simulink model "mbd_example_pwm"  (R2022b)
settings: Solver=FixedStepDiscrete  StartTime=0.0  StopTime=10.0  RelTol=1e-3  EnableMultiTasking=on
PostLoadFcn:
  | run([bdroot '_init']);
InitFcn:
  | checkModelFolder; % Optional
  | run([bdroot '_init']);
values from neighbouring files (symbols this model uses):
  T_s_LED1 = 1/LED1_Hz    (= 0.5)    [mbd_example_pwm_init.m]
  T_s_LED2 = 1/LED2_Hz    (= 1)    [mbd_example_pwm_init.m]
libraries: MbdLib_Pwm x14, MbdLib_Digital x11, MbdLib_Timer x5, MbdLib_Sys x4, MbdLib_LpTimer x4, MbdLib_Required x1
settings Model: Creator=KenYoshioka  LastModifiedBy=KenYoshioka
settings SolverCC: AutoInsertRateTranBlk=on
settings OptimizationCC: DefaultParameterBehavior=Inlined  DefaultUnderspecifiedDataType=single  EnhancedBackFolding=on  BooleansAsBitfields=on  PassReuseOutputArgsAs=Individual arguments  ZeroExternalMemoryAtStartup=off  ZeroInternalMemoryAtStartup=off  OptimizeBlockOrder=speed  DifferentSizesBufferReuse=on  EfficientTunableParamExpr=on
settings DebuggingCC: ParameterTunabilityLossMsg=error
settings HardwareCC: ProdBitPerPointer=32  ProdBitPerSizeT=32  ProdBitPerPtrDiffT=32  ProdLargestAtomicInteger=Long  ProdLargestAtomicFloat=Double  ProdWordSize=32  ProdHWDeviceType=ARM Compatible->ARM Cortex-M
settings ModelReferenceCC: EnableRefExpFcnMdlSchedulingChecks=on  ModelReferenceNumInstancesAllowed=Single
settings SFSimCC: MATLABDynamicMemAlloc=off
settings RTWCC: Description=MBD Embedded Target STM32 Cortex M4 (real-time)  SystemTargetFile=MBD_STM32_stf.tlc  TemplateMakefile=MBD_STM32.tmf  Toolchain=arm-none-eabi - v9.3.1
settings CodeAppCC: ForceParamTrailComments=on  IgnoreCustomStorageClasses=off  MaxIdLength=255  OperatorAnnotations=on  SimulinkDataObjDesc=on  SFDataObjDesc=on  InsertBlockDesc=on
settings STFCustomTargetCC: MultiwordLength=256  IncludeMdlTerminateFcn=off  CombineOutputUpdateFcns=on  CombineSignalStateStructs=on  SuppressErrorStatus=on  ERTCustomFileBanners=on  SupportContinuousTime=off  RemoveResetFunc=on  MATLABClassNameForMDSCustomization=Simulink.SoftwareTarget.ERTCustomization  UseToolchainInfoCompliant=on  SystemTargetFile=MBD_STM32_stf.tlc
settings ERTTargetCC: ParMdlRefBuildCompliant=off  CompOptLevelCompliant=off  ConcurrentExecutionCompliant=off  IncludeMdlTerminateFcn=off  CombineSignalStateStructs=on  SuppressErrorStatus=on  SupportNonInlinedSFcns=on  ModelStepFunctionPrototypeControlCompliant=off  CPPClassGenCompliant=off  ExtModeStaticAllocSize=2000  InlinedParameterPlacement=NonHierarchical  ERTCustomFileTemplate=mbd_lib_interface.tlc  MaxLineWidth=110

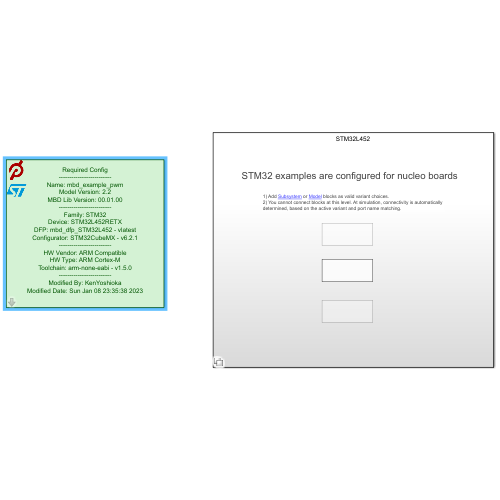
[thumbnail: Simulink's stored preview of the top-level diagram]
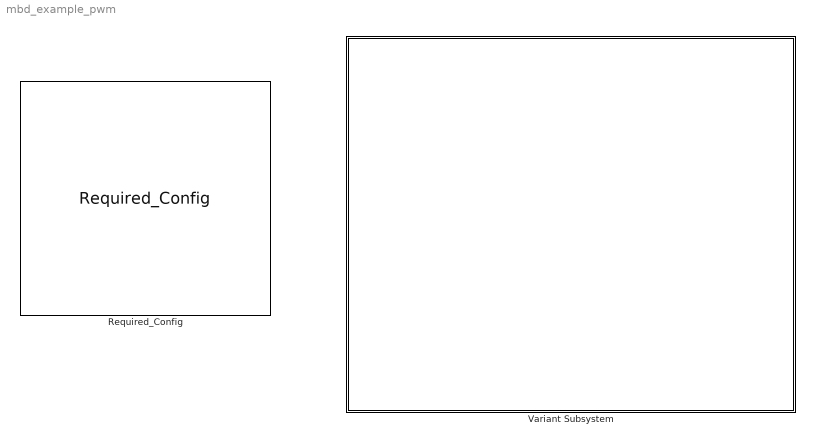
== system mbd_example_pwm ==
  Required_Config : MbdLib_Required/Required_Config  Tag=MBD_Target_Info  Param_update=1
      settings: SourceProductName=Peloton Interface Library
  Variant Subsystem : Subsystem  Variant=on

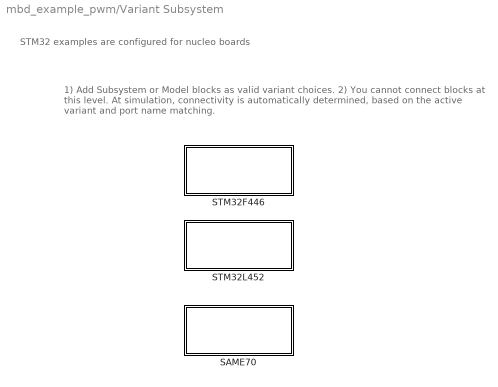
== system mbd_example_pwm/Variant Subsystem ==
  note: 1) Add Subsystem or Model blocks as valid variant choices.
      | 2) You cannot connect blocks at this level. At simulation, connectivity is automatically
      | determined, based on the active variant and port name matching.
  note: STM32 examples are configured for nucleo boards
  SAME70 : Subsystem  VariantControl=VAR_MBD_SAME70
  STM32F446 : Subsystem  VariantControl=VAR_MBD_STM32F446
  STM32L452 : Subsystem  VariantControl=VAR_MBD_STM32L452

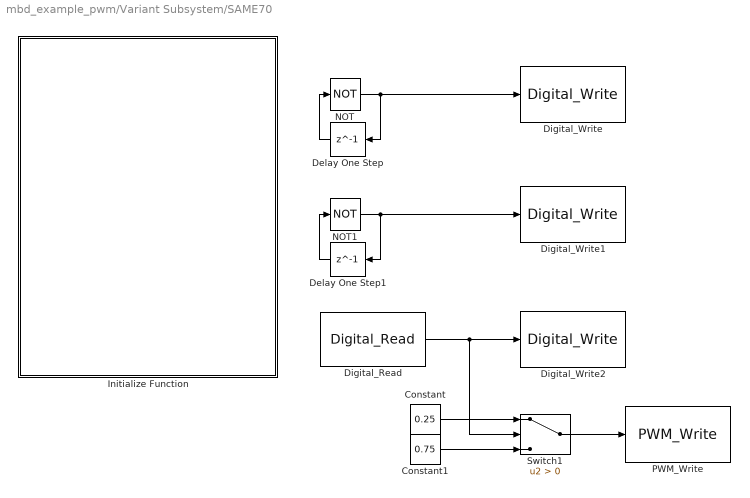
== system mbd_example_pwm/Variant Subsystem/SAME70 ==
  Constant : Constant  Value=0.25
  Constant1 : Constant  Value=0.75
  Delay One Step : Delay  DelayLength=1  SampleTime=T_s_LED1
  Delay One Step1 : Delay  DelayLength=1  SampleTime=T_s_LED2
  Digital_Read : MbdLib_Digital/Digital_Read  Param_module=D  Param_ch=28  Param_sampleTime=-1  Sim_invert=off  Sim_out=0
      settings: SourceProductName=Peloton Interface Library
  Digital_Write : MbdLib_Digital/Digital_Write  Param_module=D  Param_ch=7  Param_sampleTime=-1
      settings: SourceProductName=Peloton Interface Library
  Digital_Write1 : MbdLib_Digital/Digital_Write  Param_module=D  Param_ch=8  Param_sampleTime=-1
      settings: SourceProductName=Peloton Interface Library
  Digital_Write2 : MbdLib_Digital/Digital_Write  Param_module=D  Param_ch=9  Param_sampleTime=-1
      settings: SourceProductName=Peloton Interface Library
  Initialize Function : Subsystem  TreatAsAtomicUnit=on
  NOT : Logic  Operator=NOT  IconShape=distinctive  AllPortsSameDT=off  OutDataTypeStr=boolean
  NOT1 : Logic  Operator=NOT  IconShape=distinctive  AllPortsSameDT=off  OutDataTypeStr=boolean
  PWM_Write : MbdLib_Pwm/PWM_Write  Param_module=0  Param_ch_visible=1  Param_ch=1  Param_sync=off  Param_sampleTime=-1
      settings: SourceProductName=Peloton Interface Library
  Switch1 : Switch  Criteria=u2 > Threshold  SaturateOnIntegerOverflow=off  InputSameDT=off
  wires:
  NOT1/1 -> Digital_Write1/1, Delay One Step1/1
  NOT/1 -> Digital_Write/1, Delay One Step/1
  Delay One Step/1 -> NOT/1
  Delay One Step1/1 -> NOT1/1
  Digital_Read/1 -> Switch1/2, Digital_Write2/1
  Constant/1 -> Switch1/1
  Constant1/1 -> Switch1/3
  Switch1/1 -> PWM_Write/1

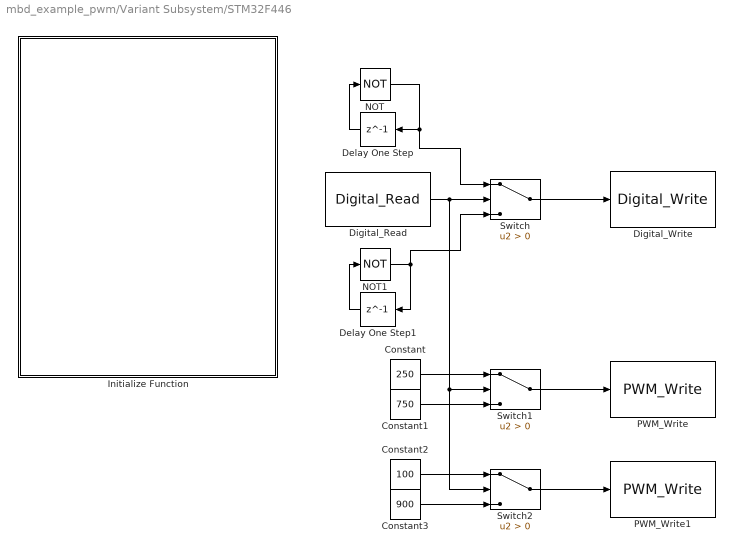
== system mbd_example_pwm/Variant Subsystem/STM32F446 ==
  Constant : Constant  Value=250
  Constant1 : Constant  Value=750
  Constant2 : Constant  Value=100
  Constant3 : Constant  Value=900
  Delay One Step : Delay  DelayLength=1  SampleTime=T_s_LED1
  Delay One Step1 : Delay  DelayLength=1  SampleTime=T_s_LED2
  Digital_Read : MbdLib_Digital/Digital_Read  Param_module=C  Param_ch=13  Param_sampleTime=-1  Sim_invert=off  Sim_out=0
      settings: SourceProductName=Peloton Interface Library
  Digital_Write : MbdLib_Digital/Digital_Write  Param_module=C  Param_ch=10  Param_sampleTime=-1
      settings: SourceProductName=Peloton Interface Library
  Initialize Function : Subsystem  TreatAsAtomicUnit=on
  NOT : Logic  Operator=NOT  IconShape=distinctive  AllPortsSameDT=off  OutDataTypeStr=boolean
  NOT1 : Logic  Operator=NOT  IconShape=distinctive  AllPortsSameDT=off  OutDataTypeStr=boolean
  PWM_Write : MbdLib_Pwm/PWM_Write  Param_module=2  Param_ch_visible=1  Param_ch=1  Param_sync=off  Param_sampleTime=-1
      settings: SourceProductName=Peloton Interface Library
  PWM_Write1 : MbdLib_Pwm/PWM_Write  Param_module=2  Param_ch_visible=2  Param_ch=2  Param_sync=off  Param_sampleTime=-1
      settings: SourceProductName=Peloton Interface Library
  Switch : Switch  Criteria=u2 > Threshold  SaturateOnIntegerOverflow=off  InputSameDT=off
  Switch1 : Switch  Criteria=u2 > Threshold  SaturateOnIntegerOverflow=off  InputSameDT=off
  Switch2 : Switch  Criteria=u2 > Threshold  SaturateOnIntegerOverflow=off  InputSameDT=off
  wires:
  NOT1/1 -> Switch/3, Delay One Step1/1
  NOT/1 -> Switch/1, Delay One Step/1
  Delay One Step/1 -> NOT/1
  Delay One Step1/1 -> NOT1/1
  Switch/1 -> Digital_Write/1
  Switch1/1 -> PWM_Write/1
  Constant/1 -> Switch1/1
  Constant1/1 -> Switch1/3
  Constant2/1 -> Switch2/1
  Constant3/1 -> Switch2/3
  Switch2/1 -> PWM_Write1/1
  Digital_Read/1 -> Switch2/2, Switch1/2, Switch/2

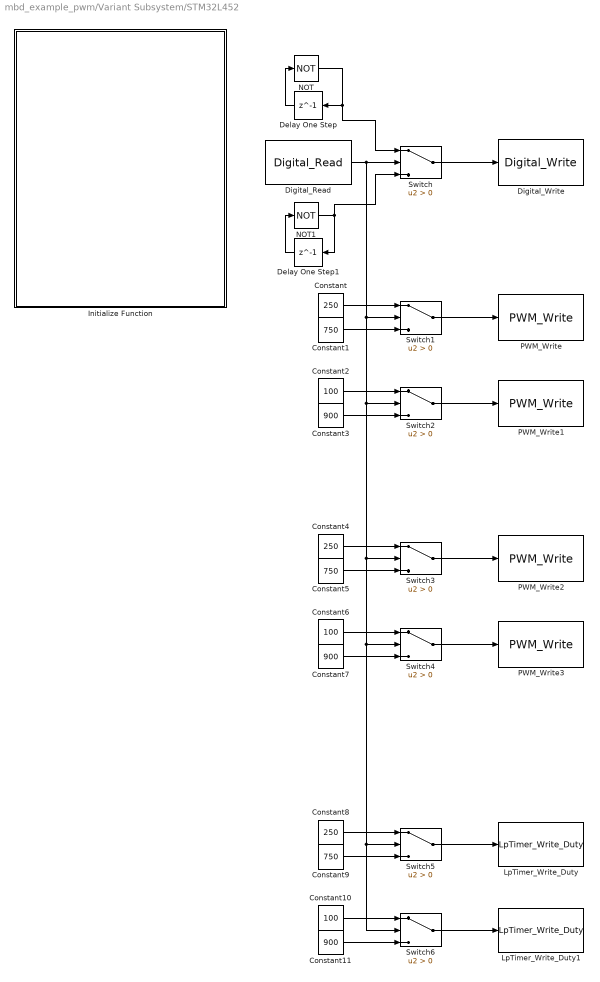
== system mbd_example_pwm/Variant Subsystem/STM32L452 ==
  Constant : Constant  Value=250
  Constant1 : Constant  Value=750
  Constant10 : Constant  Value=100
  Constant11 : Constant  Value=900
  Constant2 : Constant  Value=100
  Constant3 : Constant  Value=900
  Constant4 : Constant  Value=250
  Constant5 : Constant  Value=750
  Constant6 : Constant  Value=100
  Constant7 : Constant  Value=900
  Constant8 : Constant  Value=250
  Constant9 : Constant  Value=750
  Delay One Step : Delay  DelayLength=1  SampleTime=T_s_LED1
  Delay One Step1 : Delay  DelayLength=1  SampleTime=T_s_LED2
  Digital_Read : MbdLib_Digital/Digital_Read  Param_module=C  Param_ch=13  Param_sampleTime=-1  Sim_invert=off  Sim_out=0
      settings: SourceProductName=Peloton Interface Library
  Digital_Write : MbdLib_Digital/Digital_Write  Param_module=C  Param_ch=10  Param_sampleTime=-1
      settings: SourceProductName=Peloton Interface Library
  Initialize Function : Subsystem  TreatAsAtomicUnit=on
  LpTimer_Write_Duty : MbdLib_LpTimer/LpTimer_Write_Duty  Param_module=1  Param_sampleTime=-1
      settings: SourceProductName=Peloton Interface Library
  LpTimer_Write_Duty1 : MbdLib_LpTimer/LpTimer_Write_Duty  Param_module=2  Param_sampleTime=-1
      settings: SourceProductName=Peloton Interface Library
  NOT : Logic  Operator=NOT  IconShape=distinctive  AllPortsSameDT=off  OutDataTypeStr=boolean
  NOT1 : Logic  Operator=NOT  IconShape=distinctive  AllPortsSameDT=off  OutDataTypeStr=boolean
  PWM_Write : MbdLib_Pwm/PWM_Write  Param_module=1  Param_ch_visible=1  Param_ch=1  Param_sync=off  Param_sampleTime=-1
      settings: SourceProductName=Peloton Interface Library
  PWM_Write1 : MbdLib_Pwm/PWM_Write  Param_module=1  Param_ch_visible=2  Param_ch=2  Param_sync=off  Param_sampleTime=-1
      settings: SourceProductName=Peloton Interface Library
  PWM_Write2 : MbdLib_Pwm/PWM_Write  Param_module=2  Param_ch_visible=1  Param_ch=1  Param_sync=off  Param_sampleTime=-1
      settings: SourceProductName=Peloton Interface Library
  PWM_Write3 : MbdLib_Pwm/PWM_Write  Param_module=2  Param_ch_visible=2  Param_ch=2  Param_sync=off  Param_sampleTime=-1
      settings: SourceProductName=Peloton Interface Library
  Switch{,1..6} (7 alike) : Switch  Criteria=u2 > Threshold  SaturateOnIntegerOverflow=off  InputSameDT=off
  wires:
  NOT1/1 -> Switch/3, Delay One Step1/1
  NOT/1 -> Switch/1, Delay One Step/1
  Delay One Step/1 -> NOT/1
  Delay One Step1/1 -> NOT1/1
  Switch/1 -> Digital_Write/1
  Switch1/1 -> PWM_Write/1
  Constant/1 -> Switch1/1
  Constant1/1 -> Switch1/3
  Constant3/1 -> Switch2/3
  Constant2/1 -> Switch2/1
  Switch2/1 -> PWM_Write1/1
  Constant7/1 -> Switch4/3
  Constant6/1 -> Switch4/1
  Constant5/1 -> Switch3/3
  Constant4/1 -> Switch3/1
  Switch3/1 -> PWM_Write2/1
  Switch4/1 -> PWM_Write3/1
  Constant11/1 -> Switch6/3
  Constant8/1 -> Switch5/1
  Constant10/1 -> Switch6/1
  Digital_Read/1 -> Switch6/2, Switch5/2, Switch4/2, Switch3/2, Switch2/2, Switch1/2, Switch/2
  Constant9/1 -> Switch5/3
  Switch5/1 -> LpTimer_Write_Duty/1
  Switch6/1 -> LpTimer_Write_Duty1/1

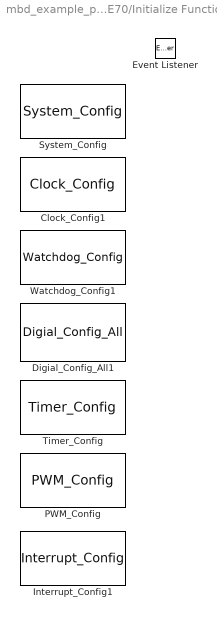
== system mbd_example_pwm/Variant Subsystem/SAME70/Initialize Function ==
  Clock_Config1 : MbdLib_Sys/Clock_Config  Priority=10  Param_frequency=Peripheral_Clock_Hz  Param_priority=10  Param_sampleTime=-1
      settings: AttributesFormatString=priority=%<priority>  SourceProductName=Peloton Interface Library
  Digial_Config_All1 : MbdLib_Digital/Digial_Config_All  Priority=30  Param_channels={ 'A', '0', 'off', '0 : input', '0 : low', '0 : none', '0 : none', '0 : low', '0 : low'; 'A', '1', 'off', '0 : input', '0 : low', '0 : none', '0 : none', '0 : low', '0 : low'; 'A', '2', 'off', '0 : input', '0 : low', '0 : none', '0 : none', '0 : low', '0 : low'; 'A', '3', 'off', '0 : input', '0 : low', '0 : none', '0 : none', '0 : low', '0 : low'; 'A', '4', 'off', '0 : input', '0 : low', '0 : none', '0 : none', '0 : low', '0 : low'; 'A', '5', 'off', '0 : input', '0 : low', '0 : none', '0 : none', '0 : low', '0 : low'; 'A', '6', 'off', '0 : input', '0 : low', '0 : none', '0 : none', '0 : low', '0 : low'; 'A', '7', 'off', '0 : input', '0 : low', '0 : none', '0 : none', '0 : low', '0 : low'; 'A', '8', 'off', '0 : input', '0 : low', '0 : none', '0 : none', '0 : low', '0 : low'; 'A', '9', 'off', '0 : input', '0 : low', '0 : none', '0 : none', '0 : low', '0 : low'; 'A', '10', 'off', '0 : input', '0 : low', '0 : none', '0 : none', '0 : low', '0 : low'; 'A', '11', 'off', '0 : input', '0 : low', '0 : none', '0 : none', '0 : low', '0 : low'; 'A', '12', 'off', '0 : input', '0 : low', '0 : none', '0 : none', '0 : low', '0 : low'; 'A', '13', 'off', '0 : input', '0 : low', '0 : none', '0 : none', '0 : low', '0 : low'; 'A', '14', 'off', '0 : input', '0 : low', '0 : none', '0 : none', '0 : low', '0 : low'; 'A', '15', 'off', '0 : input', '0 : low', '0 : none', '0 : none', '0 : low', '0 : low'; 'A', '16', 'off', '0 : input', '0 : low', '0 : none', '0 : none', '0 : low', '0 : low'; 'A', '17', 'off', '0 : input', '0 : low', '0 : none', '0 : none', '0 : low', '0 : low'; 'A', '18', 'off', '0 : input', '0 : low', '0 : none', '0 : none', '0 : low', '0 : low'; 'A', '19', 'off', '0 : input', '0 : low', '0 : none', '0 : none', '0 : low', '0 : low'; 'A', '20', 'off', '0 : input', '0 : low', '0 : none', '0 : none', '0 : low', '0 : low'; 'A', '21', 'off', '0 : input', '0 : low', '0 : none', '0 : none', '0 : low', '0 : low'; 'A', '22', 'off', '0 : input', '0 : low', '0 : none', '0 : none', '0 : low', '0 : low'; 'A', '23', 'off', '0 : input', '0 : low', '0 : none', '0 : none', '0 : low', '0 : low'; 'A', '24', 'off', '0 : input', '0 : low', '0 : none', '0 : none', '0 : low', '0 : low'; 'A', '25', 'off', '0 : input', '0 : low', '0 : none', '0 : none', '0 : low', '0 : low'; 'A', '26', 'off', '0 : input', '0 : low', '0 : none', '0 : none', '0 : low', '0 : low'; 'A', '27', 'off', '0 : input', '0 : low', '0 : none', '0 : none', '0 : low', '0 : low'; 'A', '28', 'off', '0 : input', '0 : low', '0 : none', '0 : none', '0 : low', '0 : low'; 'A', '29', 'off', '0 : input', '0 : low', '0 : none', '0 : none', '0 : low', '0 : low'; 'A', '30', 'off', '0 : input', '0 : low', '0 : none', '0 : none', '0 : low', '0 : low'; 'A', '31', 'off', '0 : input', '0 : low', '0 : none', '0 : none', '0 : low', '0 : low'; 'B', '0', 'off', '0 : input', '0 : low', '0 : none', '0 : none', '0 : low', '0 : low'; 'B', '1', 'off', '0 : input', '0 : low', '0 : none', '0 : none', '0 : low', '0 : low'; 'B', '2', 'off', '0 : input', '0 : low', '0 : none', '0 : none', '0 : low', '0 : low'; 'B', '3', 'off', '0 : input', '0 : low', '0 : none', '0 : none', '0 : low', '0 : low'; 'B', '4', 'off', '0 : input', '0 : low', '0 : none', '0 : none', '0 : low', '0 : low'; 'B', '5', 'off', '0 : input', '0 : low', '0 : none', '0 : none', '0 : low', '0 : low'; 'B', '6', 'off', '0 : input', '0 : low', '0 : none', '0 : none', '0 : low', '0 : low'; 'B', '7', 'off', '0 : input', '0 : low', '0 : none', '0 : none', '0 : low', '0 : low'; 'B', '8', 'off', '0 : input', '0 : low', '0 : none', '0 : none', '0 : low', '0 : low'; 'B', '9', 'off', '0 : input', '0 : low', '0 : none', '0 : none', '0 : low', '0 : low'; 'B', '10', 'off', '0 : input', '0 : low', '0 : none', '0 : none', '0 : low', '0 : low'; 'B', '11', 'off', '0 : input', '0 : low', '0 : none', '0 : none', '0 : low', '0 : low'; 'B', '12', 'off', '0 : input', '0 : low', '0 : none', '0 : none', '0 : low', '0 : low'; 'B', '13', 'off', '0 : input', '0 : low', '0 : none', '0 : none', '0 : low', '0 : low'; 'C', '0', 'off', '0 : input', '0 : low', '0 : none', '0 : none', '0 : low', '0 : low'; 'C', '1', 'off', '0 : input', '0 : low', '0 : none', '0 : none', '0 : low', '0 : low'; 'C', '2', 'off', '0 : input', '0 : low', '0 : none', '0 : none', '0 : low', '0 : low'; 'C', '3', 'off', '0 : input', '0 : low', '0 : none', '0 : none', '0 : low', '0 : low'; 'C', '4', 'off', '0 : input', '0 : low', '0 : none', '0 : none', '0 : low', '0 : low'; 'C', '5', 'off', '0 : input', '0 : low', '0 : none', '0 : none', '0 : low', '0 : low'; 'C', '6', 'off', '0 : input', '0 : low', '0 : none', '0 : none', '0 : low', '0 : low'; 'C', '7', 'off', '0 : input', '0 : low', '0 : none', '0 : none', '0 : low', '0 : low'; 'C', '8', 'off', '0 : input', '0 : low', '0 : none', '0 : none', '0 : low', '0 : low'; 'C', '9', 'off', '0 : input', '0 : low', '0 : none', '0 : none', '0 : low', '0 : low'; 'C', '10', 'off', '0 : input', '0 : low', '0 : none', '0 : none', '0 : low', '0 : low'; 'C', '11', 'off', '0 : input', '0 : low', '0 : none', '0 : none', '0 : low', '0 : low'; 'C', '12', 'off', '0 : input', '0 : low', '0 : none', '0 : none', '0 : low', '0 : low'; 'C', '13', 'off', '0 : input', '0 : low', '0 : none', '0 : none', '0 : low', '0 : low'; 'C', '14', 'off', '0 : input', '0 : low', '0 : none', '0 : none', '0 : low', '0 : low'; 'C', '15', 'off', '0 : input', '0 : low', '0 : none', '0 : none', '0 : low', '0 : low'; 'C', '16', 'off', '0 : input', '0 : low', '0 : none', '0 : none', '0 : low', '0 : low'; 'C', '17', 'off', '0 : input', '0 : low', '0 : none', '0 : none', '0 : low', '0 : low'; 'C', '18', 'off', '0 : input', '0 : low', '0 : none', '0 : none', '0 : low', '0 : low'; 'C', '19', 'off', '0 : input', '0 : low', '0 : none', '0 : none', '0 : low', '0 : low'; 'C', '20', 'off', '0 : input', '0 : low', '0 : none', '0 : none', '0 : low', '0 : low'; 'C', '21', 'off', '0 : input', '0 : low', '0 : none', '0 : none', '0 : low', '0 : low'; 'C', '22', 'off', '0 : input', '0 : low', '0 : none', '0 : none', '0 : low', '0 : low'; 'C', '23', 'off', '0 : input', '0 : low', '0 : none', '0 : none', '0 : low', '0 : low'; 'C', '24', 'off', '0 : input', '0 : low', '0 : none', '0 : none', '0 : low', '0 : low'; 'C', '25', 'off', '0 : input', '0 : low', '0 : none', '0 : none', '0 : low', '0 : low'; 'C', '26', 'off', '0 : input', '0 : low', '0 : none', '0 : none', '0 : low', '0 : low'; 'C', '27', 'off', '0 : input', '0 : low', '0 : none', '0 : none', '0 : low', '0 : low'; 'C', '28', 'off', '0 : input', '0 : low', '0 : none', '0 : none', '0 : low', '0 : low'; 'C', '29', 'off', '0 : input', '0 : low', '0 : none', '0 : none', '0 : low', '0 : low'; 'C', '30', 'off', '0 : input', '0 : low', '0 : none', '0 : none', '0 : low', '0 : low'; 'C', '31', 'off', '0 : input', '0 : low', '0 : none', '0 : none', '0 : low', '0 : low'; 'D', '0', 'off', '0 : input', '0 : low', '0 : none', '0 : none', '0 : low', '0 : low'; 'D', '1', 'off', '0 : input', '0 : low', '0 : none', '0 : none', '0 : low', '0 : low'; 'D', '2', 'off', '0 : input', '0 : low', '0 : none', '0 : none', '0 : low', '0 : low'; 'D', '3', 'off', '0 : input', '0 : low', '0 : none', '0 : none', '0 : low', '0 : low'; 'D', '4', 'off', '0 : input', '0 : low', '0 : none', '0 : none', '0 : low', '0 : low'; 'D', '5', 'off', '0 : input', '0 : low', '0 : none', '0 : none', '0 : low', '0 : low'; 'D', '6', 'off', '0 : input', '0 : low', '0 : none', '0 : none', '0 : low', '0 : low'; 'D', '7', 'on', '1 : output', '0 : low', '0 : none', '0 : none', '0 : low', '0 : low'; 'D', '8', 'on', '1 : output', '0 : low', '0 : none', '0 : none', '0 : low', '0 : low'; 'D', '9', 'on', '1 : output', '0 : low', '0 : none', '0 : none', '0 : low', '0 : low'; 'D', '10', 'off', '0 : input', '0 : low', '0 : none', '0 : none', '0 : low', '0 : low'; 'D', '11', 'off', '0 : input', '0 : low', '0 : none', '0 : none', '0 : low', '0 : low'; 'D', '12', 'off', '0 : input', '0 : low', '0 : none', '0 : none', '0 : low', '0 : low'; 'D', '13', 'off', '0 : input', '0 : low', '0 : none', '0 : none', '0 : low', '0 : low'; 'D', '14', 'off', '0 : input', '0 : low', '0 : none', '0 : none', '0 : low', '0 : low'; 'D', '15', 'off', '0 : input', '0 : low', '0 : none', '0 : none', '0 : low', '0 : low'; 'D', '16', 'off', '0 : input', '0 : low', '0 : none', '0 : none', '0 : low', '0 : low'; 'D', '17', 'off', '0 : input', '0 : low', '0 : none', '0 : none', '0 : low', '0 : low'; 'D', '18', 'off', '0 : input', '0 : low', '0 : none', '0 : none', '0 : low', '0 : low'; 'D', '19', 'off', '0 : input', '0 : low', '0 : none', '0 : none', '0 : low', '0 : low'; 'D', '20', 'off', '0 : input', '0 : low', '0 : none', '0 : none', '0 : low', '0 : low'; 'D', '21', 'off', '0 : input', '0 : low', '0 : none', '0 : none', '0 : low', '0 : low'; 'D', '22', 'off', '0 : input', '0 : low', '0 : none', '0 : none', '0 : low', '0 : low'; 'D', '23', 'off', '0 : input', '0 : low', '0 : none', '0 : none', '0 : low', '0 : low'; 'D', '24', 'off', '0 : input', '0 : low', '0 : none', '0 : none', '0 : low', '0 : low'; 'D', '25', 'off', '0 : input', '0 : low', '0 : none', '0 : none', '0 : low', '0 : low'; 'D', '26', 'off', '0 : input', '0 : low', '0 : none', '0 : none', '0 : low', '0 : low'; 'D', '27', 'off', '0 : input', '0 : low', '0 : none', '0 : none', '0 : low', '0 : low'; 'D', '28', 'off', '0 : input', '0 : low', '0 : none', '0 : none', '0 : low', '0 : low'; 'D', '29', 'off', '0 : input', '0 : low', '0 : none', '0 : none', '0 : low', '0 : low'; 'D', '30', 'off', '0 : input', '0 : low', '0 : none', '0 : none', '0 : low', '0 : low'; 'D', '31', 'off', '0 : input', '0 : low', '0 : none', '0 : none', '0 : low', '0 : low'; 'E', '0', 'off', '0 : input', '0 : low', '0 : none', '0 : none', '0 : low', '0 : low'; 'E', '1', 'off', '0 : input', '0 : low', '0 : none', '0 : none', '0 : low', '0 : low'; 'E', '2', 'off', '0 : input', '0 : low', '0 : none', '0 : none', '0 : low', '0 : low'; 'E', '3', 'off', '0 : input', '0 : low', '0 : none', '0 : none', '0 : low', '0 : low'; 'E', '4', 'off', '0 : input', '0 : low', '0 : none', '0 : none', '0 : low', '0 : low'; 'E', '5', 'off', '0 : input', '0 : low', '0 : none', '0 : none', '0 : low', '0 : low' }  Param_priority=30  Param_sampleTime=-1
      settings: AttributesFormatString=priority=%<priority>  SourceProductName=Peloton Interface Library
  Event Listener : EventListener  DisableCoverage=on  EventName=reset
  Interrupt_Config1 : MbdLib_Sys/Interrupt_Config  Priority=120  Param_priority=120  Param_sampleTime=-1
      settings: AttributesFormatString=priority=%<priority>  SourceProductName=Peloton Interface Library
  PWM_Config : MbdLib_Pwm/PWM_Config  Priority=110  Param_module=0  Param_clksrc=0  Param_period=0  Param_channels={ '0', 'off', '0', '0', 'off'; '1', 'off', '0', '0', 'off'; '2', 'off', '0', '0', 'off'; '3', 'off', '0', '0', 'off' }  Param_priority=110  Param_sampleTime=-1
      settings: AttributesFormatString=priority=%<priority>  SourceProductName=Peloton Interface Library
  System_Config : MbdLib_Sys/System_Config  Priority=0  Param_priority=0  Param_sampleTime=-1
      settings: AttributesFormatString=priority=%<priority>  SourceProductName=Peloton Interface Library
  Timer_Config : MbdLib_Timer/Timer_Config  Priority=100  Param_update=1  Param_module=2  Param_step=0  Param_period=LED1_period_cycles  Param_divider=0  Param_step0=0  Param_clksrc0=2  Param_period0=LED1_period_cycles  Param_divider0=0  Param_step1=1  Param_clksrc1=2  Param_period1=LED2_period_cycles  Param_divider1=0  Param_step2=-1  Param_clksrc2=0  Param_period2=0  Param_divider2=0  Param_priority=100  Param_sampleTime=-1
      settings: AttributesFormatString=priority=%<priority>  SourceProductName=Peloton Interface Library
  Watchdog_Config1 : MbdLib_Sys/Watchdog_Config  Priority=20  Param_enable=off  Param_priority=20  Param_sampleTime=-1
      settings: AttributesFormatString=priority=%<priority>  SourceProductName=Peloton Interface Library

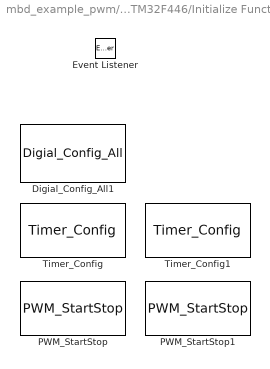
== system mbd_example_pwm/Variant Subsystem/STM32F446/Initialize Function ==
  Digial_Config_All1 : MbdLib_Digital/Digial_Config_All  Priority=30  Param_channels={ 'A', '0', 'off', '0 : input', '0 : low', '0 : none', '0 : none', '0 : low', '0 : low'; 'A', '1', 'off', '0 : input', '0 : low', '0 : none', '0 : none', '0 : low', '0 : low'; 'A', '2', 'off', '0 : input', '0 : low', '0 : none', '0 : none', '0 : low', '0 : low'; 'A', '3', 'off', '0 : input', '0 : low', '0 : none', '0 : none', '0 : low', '0 : low'; 'A', '4', 'off', '0 : input', '0 : low', '0 : none', '0 : none', '0 : low', '0 : low'; 'A', '5', 'off', '0 : input', '0 : low', '0 : none', '0 : none', '0 : low', '2 : high'; 'A', '6', 'off', '0 : input', '0 : low', '0 : none', '0 : none', '0 : low', '0 : low'; 'A', '7', 'off', '0 : input', '0 : low', '0 : none', '0 : none', '0 : low', '0 : low'; 'A', '8', 'off', '0 : input', '0 : low', '0 : none', '0 : none', '0 : low', '0 : low'; 'A', '9', 'off', '0 : input', '0 : low', '0 : none', '0 : none', '0 : low', '0 : low'; 'A', '10', 'off', '0 : input', '0 : low', '0 : none', '0 : none', '0 : low', '0 : low'; 'A', '11', 'off', '0 : input', '0 : low', '0 : none', '0 : none', '0 : low', '0 : low'; 'A', '12', 'off', '0 : input', '0 : low', '0 : none', '0 : none', '0 : low', '0 : low'; 'A', '13', 'off', '0 : input', '0 : low', '0 : none', '0 : none', '0 : low', '0 : low'; 'A', '14', 'off', '0 : input', '0 : low', '0 : none', '0 : none', '0 : low', '0 : low'; 'A', '15', 'off', '0 : input', '0 : low', '0 : none', '0 : none', '0 : low', '0 : low'; 'A', '16', 'off', '0 : input', '0 : low', '0 : none', '0 : none', '0 : low', '0 : low'; 'A', '17', 'off', '0 : input', '0 : low', '0 : none', '0 : none', '0 : low', '0 : low'; 'A', '18', 'off', '0 : input', '0 : low', '0 : none', '0 : none', '0 : low', '0 : low'; 'A', '19', 'off', '0 : input', '0 : low', '0 : none', '0 : none', '0 : low', '0 : low'; 'A', '20', 'off', '0 : input', '0 : low', '0 : none', '0 : none', '0 : low', '0 : low'; 'A', '21', 'off', '0 : input', '0 : low', '0 : none', '0 : none', '0 : low', '0 : low'; 'A', '22', 'off', '0 : input', '0 : low', '0 : none', '0 : none', '0 : low', '0 : low'; 'A', '23', 'off', '0 : input', '0 : low', '0 : none', '0 : none', '0 : low', '0 : low'; 'A', '24', 'off', '0 : input', '0 : low', '0 : none', '0 : none', '0 : low', '0 : low'; 'A', '25', 'off', '0 : input', '0 : low', '0 : none', '0 : none', '0 : low', '0 : low'; 'A', '26', 'off', '0 : input', '0 : low', '0 : none', '0 : none', '0 : low', '0 : low'; 'A', '27', 'off', '0 : input', '0 : low', '0 : none', '0 : none', '0 : low', '0 : low'; 'A', '28', 'off', '0 : input', '0 : low', '0 : none', '0 : none', '0 : low', '0 : low'; 'A', '29', 'off', '0 : input', '0 : low', '0 : none', '0 : none', '0 : low', '0 : low'; 'A', '30', 'off', '0 : input', '0 : low', '0 : none', '0 : none', '0 : low', '0 : low'; 'A', '31', 'off', '0 : input', '0 : low', '0 : none', '0 : none', '0 : low', '0 : low'; 'B', '0', 'off', '0 : input', '0 : low', '0 : none', '0 : none', '0 : low', '0 : low'; 'B', '1', 'off', '0 : input', '0 : low', '0 : none', '0 : none', '0 : low', '0 : low'; 'B', '2', 'off', '0 : input', '0 : low', '0 : none', '0 : none', '0 : low', '0 : low'; 'B', '3', 'off', '0 : input', '0 : low', '0 : none', '0 : none', '0 : low', '0 : low'; 'B', '4', 'off', '0 : input', '0 : low', '0 : none', '0 : none', '0 : low', '0 : low'; 'B', '5', 'off', '0 : input', '0 : low', '0 : none', '0 : none', '0 : low', '0 : low'; 'B', '6', 'off', '0 : input', '0 : low', '0 : none', '0 : none', '0 : low', '0 : low'; 'B', '7', 'off', '0 : input', '0 : low', '0 : none', '0 : none', '0 : low', '0 : low'; 'B', '8', 'off', '0 : input', '0 : low', '0 : none', '0 : none', '0 : low', '0 : low'; 'B', '9', 'off', '0 : input', '0 : low', '0 : none', '0 : none', '0 : low', '0 : low'; 'B', '10', 'off', '0 : input', '0 : low', '0 : none', '0 : none', '0 : low', '0 : low'; 'B', '11', 'off', '0 : input', '0 : low', '0 : none', '0 : none', '0 : low', '0 : low'; 'B', '12', 'off', '0 : input', '0 : low', '0 : none', '0 : none', '0 : low', '0 : low'; 'B', '13', 'off', '0 : input', '0 : low', '0 : none', '0 : none', '0 : low', '0 : low'; 'C', '0', 'off', '0 : input', '0 : low', '0 : none', '0 : none', '0 : low', '0 : low'; 'C', '1', 'off', '0 : input', '0 : low', '0 : none', '0 : none', '0 : low', '0 : low'; 'C', '2', 'off', '0 : input', '0 : low', '0 : none', '0 : none', '0 : low', '0 : low'; 'C', '3', 'off', '0 : input', '0 : low', '0 : none', '0 : none', '0 : low', '0 : low'; 'C', '4', 'off', '0 : input', '0 : low', '0 : none', '0 : none', '0 : low', '0 : low'; 'C', '5', 'off', '0 : input', '0 : low', '0 : none', '0 : none', '0 : low', '0 : low'; 'C', '6', 'off', '0 : input', '0 : low', '0 : none', '0 : none', '0 : low', '0 : low'; 'C', '7', 'off', '0 : input', '0 : low', '0 : none', '0 : none', '0 : low', '0 : low'; 'C', '8', 'off', '0 : input', '0 : low', '0 : none', '0 : none', '0 : low', '0 : low'; 'C', '9', 'off', '0 : input', '0 : low', '0 : none', '0 : none', '0 : low', '0 : low'; 'C', '10', 'on', '1 : output', '0 : low', '0 : none', '0 : none', '0 : low', '0 : low'; 'C', '11', 'off', '0 : input', '0 : low', '0 : none', '0 : none', '0 : low', '0 : low'; 'C', '12', 'off', '0 : input', '0 : low', '0 : none', '0 : none', '0 : low', '0 : low'; 'C', '13', 'on', '0 : input', '0 : low', '0 : none', '1 : pullup', '0 : low', '0 : low'; 'C', '14', 'off', '0 : input', '0 : low', '0 : none', '0 : none', '0 : low', '0 : low'; 'C', '15', 'off', '0 : input', '0 : low', '0 : none', '0 : none', '0 : low', '0 : low'; 'C', '16', 'off', '0 : input', '0 : low', '0 : none', '0 : none', '0 : low', '0 : low'; 'C', '17', 'off', '0 : input', '0 : low', '0 : none', '0 : none', '0 : low', '0 : low'; 'C', '18', 'off', '0 : input', '0 : low', '0 : none', '0 : none', '0 : low', '0 : low'; 'C', '19', 'off', '0 : input', '0 : low', '0 : none', '0 : none', '0 : low', '0 : low'; 'C', '20', 'off', '0 : input', '0 : low', '0 : none', '0 : none', '0 : low', '0 : low'; 'C', '21', 'off', '0 : input', '0 : low', '0 : none', '0 : none', '0 : low', '0 : low'; 'C', '22', 'off', '0 : input', '0 : low', '0 : none', '0 : none', '0 : low', '0 : low'; 'C', '23', 'off', '0 : input', '0 : low', '0 : none', '0 : none', '0 : low', '0 : low'; 'C', '24', 'off', '0 : input', '0 : low', '0 : none', '0 : none', '0 : low', '0 : low'; 'C', '25', 'off', '0 : input', '0 : low', '0 : none', '0 : none', '0 : low', '0 : low'; 'C', '26', 'off', '0 : input', '0 : low', '0 : none', '0 : none', '0 : low', '0 : low'; 'C', '27', 'off', '0 : input', '0 : low', '0 : none', '0 : none', '0 : low', '0 : low'; 'C', '28', 'off', '0 : input', '0 : low', '0 : none', '0 : none', '0 : low', '0 : low'; 'C', '29', 'off', '0 : input', '0 : low', '0 : none', '0 : none', '0 : low', '0 : low'; 'C', '30', 'off', '0 : input', '0 : low', '0 : none', '0 : none', '0 : low', '0 : low'; 'C', '31', 'off', '0 : input', '0 : low', '0 : none', '0 : none', '0 : low', '0 : low'; 'D', '0', 'off', '0 : input', '0 : low', '0 : none', '0 : none', '0 : low', '0 : low'; 'D', '1', 'off', '0 : input', '0 : low', '0 : none', '0 : none', '0 : low', '0 : low'; 'D', '2', 'off', '0 : input', '0 : low', '0 : none', '0 : none', '0 : low', '0 : low'; 'D', '3', 'off', '0 : input', '0 : low', '0 : none', '0 : none', '0 : low', '0 : low'; 'D', '4', 'off', '0 : input', '0 : low', '0 : none', '0 : none', '0 : low', '0 : low'; 'D', '5', 'off', '0 : input', '0 : low', '0 : none', '0 : none', '0 : low', '0 : low'; 'D', '6', 'off', '0 : input', '0 : low', '0 : none', '0 : none', '0 : low', '0 : low'; 'D', '7', 'off', '0 : input', '0 : low', '0 : none', '0 : none', '0 : low', '0 : low'; 'D', '8', 'off', '0 : input', '0 : low', '0 : none', '0 : none', '0 : low', '0 : low'; 'D', '9', 'off', '0 : input', '0 : low', '0 : none', '0 : none', '0 : low', '0 : low'; 'D', '10', 'off', '0 : input', '0 : low', '0 : none', '0 : none', '0 : low', '0 : low'; 'D', '11', 'off', '0 : input', '0 : low', '0 : none', '0 : none', '0 : low', '0 : low'; 'D', '12', 'off', '0 : input', '0 : low', '0 : none', '0 : none', '0 : low', '0 : low'; 'D', '13', 'off', '0 : input', '0 : low', '0 : none', '0 : none', '0 : low', '0 : low'; 'D', '14', 'off', '0 : input', '0 : low', '0 : none', '0 : none', '0 : low', '0 : low'; 'D', '15', 'off', '0 : input', '0 : low', '0 : none', '0 : none', '0 : low', '0 : low'; 'D', '16', 'off', '0 : input', '0 : low', '0 : none', '0 : none', '0 : low', '0 : low'; 'D', '17', 'off', '0 : input', '0 : low', '0 : none', '0 : none', '0 : low', '0 : low'; 'D', '18', 'off', '0 : input', '0 : low', '0 : none', '0 : none', '0 : low', '0 : low'; 'D', '19', 'off', '0 : input', '0 : low', '0 : none', '0 : none', '0 : low', '0 : low'; 'D', '20', 'off', '0 : input', '0 : low', '0 : none', '0 : none', '0 : low', '0 : low'; 'D', '21', 'off', '0 : input', '0 : low', '0 : none', '0 : none', '0 : low', '0 : low'; 'D', '22', 'off', '0 : input', '0 : low', '0 : none', '0 : none', '0 : low', '0 : low'; 'D', '23', 'off', '0 : input', '0 : low', '0 : none', '0 : none', '0 : low', '0 : low'; 'D', '24', 'off', '0 : input', '0 : low', '0 : none', '0 : none', '0 : low', '0 : low'; 'D', '25', 'off', '0 : input', '0 : low', '0 : none', '0 : none', '0 : low', '0 : low'; 'D', '26', 'off', '0 : input', '0 : low', '0 : none', '0 : none', '0 : low', '0 : low'; 'D', '27', 'off', '0 : input', '0 : low', '0 : none', '0 : none', '0 : low', '0 : low'; 'D', '28', 'off', '0 : input', '0 : low', '0 : none', '0 : none', '0 : low', '0 : low'; 'D', '29', 'off', '0 : input', '0 : low', '0 : none', '0 : none', '0 : low', '0 : low'; 'D', '30', 'off', '0 : input', '0 : low', '0 : none', '0 : none', '0 : low', '0 : low'; 'D', '31', 'off', '0 : input', '0 : low', '0 : none', '0 : none', '0 : low', '0 : low'; 'E', '0', 'off', '0 : input', '0 : low', '0 : none', '0 : none', '0 : low', '0 : low'; 'E', '1', 'off', '0 : input', '0 : low', '0 : none', '0 : none', '0 : low', '0 : low'; 'E', '2', 'off', '0 : input', '0 : low', '0 : none', '0 : none', '0 : low', '0 : low'; 'E', '3', 'off', '0 : input', '0 : low', '0 : none', '0 : none', '0 : low', '0 : low'; 'E', '4', 'off', '0 : input', '0 : low', '0 : none', '0 : none', '0 : low', '0 : low'; 'E', '5', 'off', '0 : input', '0 : low', '0 : none', '0 : none', '0 : low', '0 : low' }  Param_priority=30  Param_sampleTime=-1
      settings: AttributesFormatString=priority=%<priority>  SourceProductName=Peloton Interface Library
  Event Listener : EventListener  DisableCoverage=on  EventName=reset
  PWM_StartStop : MbdLib_Pwm/PWM_StartStop  Priority=120  Param_module=2  Param_ch=1  Param_action=Start  Param_priority=120  Param_sampleTime=-1
      settings: AttributesFormatString=priority=%<priority>  SourceProductName=Peloton Interface Library
  PWM_StartStop1 : MbdLib_Pwm/PWM_StartStop  Priority=120  Param_module=2  Param_ch=2  Param_action=Start  Param_priority=120  Param_sampleTime=-1
      settings: AttributesFormatString=priority=%<priority>  SourceProductName=Peloton Interface Library
  Timer_Config : MbdLib_Timer/Timer_Config  Priority=100  Param_update=1  Param_module=1  Param_step=0  Param_period=LED1_period_cycles  Param_divider=LED1_clock_divider  Param_step0=0  Param_clksrc0=0  Param_period0=LED1_period_cycles  Param_divider0=LED1_clock_divider  Param_step1=-1  Param_clksrc1=0  Param_period1=0  Param_divider1=0  Param_step2=-1  Param_clksrc2=0  Param_period2=0  Param_divider2=0  Param_priority=100  Param_sampleTime=-1
      settings: AttributesFormatString=priority=%<priority>  SourceProductName=Peloton Interface Library
  Timer_Config1 : MbdLib_Timer/Timer_Config  Priority=101  Param_update=1  Param_module=6  Param_step=1  Param_period=LED2_period_cycles  Param_divider=LED2_clock_divider  Param_step0=1  Param_clksrc0=0  Param_period0=LED2_period_cycles  Param_divider0=LED2_clock_divider  Param_step1=-1  Param_clksrc1=0  Param_period1=0  Param_divider1=0  Param_step2=-1  Param_clksrc2=0  Param_period2=0  Param_divider2=0  Param_priority=101  Param_sampleTime=-1
      settings: AttributesFormatString=priority=%<priority>  SourceProductName=Peloton Interface Library

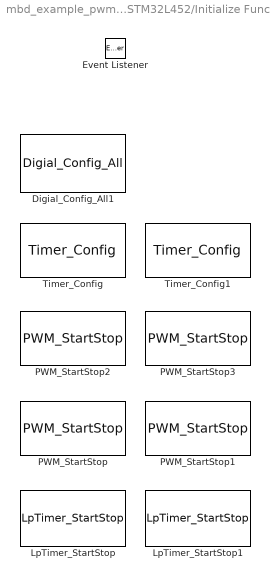
== system mbd_example_pwm/Variant Subsystem/STM32L452/Initialize Function ==
  Digial_Config_All1 : MbdLib_Digital/Digial_Config_All  Priority=30  Param_channels={ 'A', '0', 'off', '0 : input', '0 : low', '0 : none', '0 : none', '0 : low', '0 : low'; 'A', '1', 'off', '0 : input', '0 : low', '0 : none', '0 : none', '0 : low', '0 : low'; 'A', '2', 'off', '0 : input', '0 : low', '0 : none', '0 : none', '0 : low', '0 : low'; 'A', '3', 'off', '0 : input', '0 : low', '0 : none', '0 : none', '0 : low', '0 : low'; 'A', '4', 'off', '0 : input', '0 : low', '0 : none', '0 : none', '0 : low', '0 : low'; 'A', '5', 'off', '0 : input', '0 : low', '0 : none', '0 : none', '0 : low', '2 : high'; 'A', '6', 'off', '0 : input', '0 : low', '0 : none', '0 : none', '0 : low', '0 : low'; 'A', '7', 'off', '0 : input', '0 : low', '0 : none', '0 : none', '0 : low', '0 : low'; 'A', '8', 'off', '0 : input', '0 : low', '0 : none', '0 : none', '0 : low', '0 : low'; 'A', '9', 'off', '0 : input', '0 : low', '0 : none', '0 : none', '0 : low', '0 : low'; 'A', '10', 'off', '0 : input', '0 : low', '0 : none', '0 : none', '0 : low', '0 : low'; 'A', '11', 'off', '0 : input', '0 : low', '0 : none', '0 : none', '0 : low', '0 : low'; 'A', '12', 'off', '0 : input', '0 : low', '0 : none', '0 : none', '0 : low', '0 : low'; 'A', '13', 'off', '0 : input', '0 : low', '0 : none', '0 : none', '0 : low', '0 : low'; 'A', '14', 'off', '0 : input', '0 : low', '0 : none', '0 : none', '0 : low', '0 : low'; 'A', '15', 'off', '0 : input', '0 : low', '0 : none', '0 : none', '0 : low', '0 : low'; 'A', '16', 'off', '0 : input', '0 : low', '0 : none', '0 : none', '0 : low', '0 : low'; 'A', '17', 'off', '0 : input', '0 : low', '0 : none', '0 : none', '0 : low', '0 : low'; 'A', '18', 'off', '0 : input', '0 : low', '0 : none', '0 : none', '0 : low', '0 : low'; 'A', '19', 'off', '0 : input', '0 : low', '0 : none', '0 : none', '0 : low', '0 : low'; 'A', '20', 'off', '0 : input', '0 : low', '0 : none', '0 : none', '0 : low', '0 : low'; 'A', '21', 'off', '0 : input', '0 : low', '0 : none', '0 : none', '0 : low', '0 : low'; 'A', '22', 'off', '0 : input', '0 : low', '0 : none', '0 : none', '0 : low', '0 : low'; 'A', '23', 'off', '0 : input', '0 : low', '0 : none', '0 : none', '0 : low', '0 : low'; 'A', '24', 'off', '0 : input', '0 : low', '0 : none', '0 : none', '0 : low', '0 : low'; 'A', '25', 'off', '0 : input', '0 : low', '0 : none', '0 : none', '0 : low', '0 : low'; 'A', '26', 'off', '0 : input', '0 : low', '0 : none', '0 : none', '0 : low', '0 : low'; 'A', '27', 'off', '0 : input', '0 : low', '0 : none', '0 : none', '0 : low', '0 : low'; 'A', '28', 'off', '0 : input', '0 : low', '0 : none', '0 : none', '0 : low', '0 : low'; 'A', '29', 'off', '0 : input', '0 : low', '0 : none', '0 : none', '0 : low', '0 : low'; 'A', '30', 'off', '0 : input', '0 : low', '0 : none', '0 : none', '0 : low', '0 : low'; 'A', '31', 'off', '0 : input', '0 : low', '0 : none', '0 : none', '0 : low', '0 : low'; 'B', '0', 'off', '0 : input', '0 : low', '0 : none', '0 : none', '0 : low', '0 : low'; 'B', '1', 'off', '0 : input', '0 : low', '0 : none', '0 : none', '0 : low', '0 : low'; 'B', '2', 'off', '0 : input', '0 : low', '0 : none', '0 : none', '0 : low', '0 : low'; 'B', '3', 'off', '0 : input', '0 : low', '0 : none', '0 : none', '0 : low', '0 : low'; 'B', '4', 'off', '0 : input', '0 : low', '0 : none', '0 : none', '0 : low', '0 : low'; 'B', '5', 'off', '0 : input', '0 : low', '0 : none', '0 : none', '0 : low', '0 : low'; 'B', '6', 'off', '0 : input', '0 : low', '0 : none', '0 : none', '0 : low', '0 : low'; 'B', '7', 'off', '0 : input', '0 : low', '0 : none', '0 : none', '0 : low', '0 : low'; 'B', '8', 'off', '0 : input', '0 : low', '0 : none', '0 : none', '0 : low', '0 : low'; 'B', '9', 'off', '0 : input', '0 : low', '0 : none', '0 : none', '0 : low', '0 : low'; 'B', '10', 'off', '0 : input', '0 : low', '0 : none', '0 : none', '0 : low', '0 : low'; 'B', '11', 'off', '0 : input', '0 : low', '0 : none', '0 : none', '0 : low', '0 : low'; 'B', '12', 'off', '0 : input', '0 : low', '0 : none', '0 : none', '0 : low', '0 : low'; 'B', '13', 'off', '0 : input', '0 : low', '0 : none', '0 : none', '0 : low', '0 : low'; 'C', '0', 'off', '0 : input', '0 : low', '0 : none', '0 : none', '0 : low', '0 : low'; 'C', '1', 'off', '0 : input', '0 : low', '0 : none', '0 : none', '0 : low', '0 : low'; 'C', '2', 'off', '0 : input', '0 : low', '0 : none', '0 : none', '0 : low', '0 : low'; 'C', '3', 'off', '0 : input', '0 : low', '0 : none', '0 : none', '0 : low', '0 : low'; 'C', '4', 'off', '0 : input', '0 : low', '0 : none', '0 : none', '0 : low', '0 : low'; 'C', '5', 'off', '0 : input', '0 : low', '0 : none', '0 : none', '0 : low', '0 : low'; 'C', '6', 'off', '0 : input', '0 : low', '0 : none', '0 : none', '0 : low', '0 : low'; 'C', '7', 'off', '0 : input', '0 : low', '0 : none', '0 : none', '0 : low', '0 : low'; 'C', '8', 'off', '0 : input', '0 : low', '0 : none', '0 : none', '0 : low', '0 : low'; 'C', '9', 'off', '0 : input', '0 : low', '0 : none', '0 : none', '0 : low', '0 : low'; 'C', '10', 'on', '1 : output', '0 : low', '0 : none', '0 : none', '0 : low', '0 : low'; 'C', '11', 'off', '0 : input', '0 : low', '0 : none', '0 : none', '0 : low', '0 : low'; 'C', '12', 'off', '0 : input', '0 : low', '0 : none', '0 : none', '0 : low', '0 : low'; 'C', '13', 'on', '0 : input', '0 : low', '0 : none', '1 : pullup', '0 : low', '0 : low'; 'C', '14', 'off', '0 : input', '0 : low', '0 : none', '0 : none', '0 : low', '0 : low'; 'C', '15', 'off', '0 : input', '0 : low', '0 : none', '0 : none', '0 : low', '0 : low'; 'C', '16', 'off', '0 : input', '0 : low', '0 : none', '0 : none', '0 : low', '0 : low'; 'C', '17', 'off', '0 : input', '0 : low', '0 : none', '0 : none', '0 : low', '0 : low'; 'C', '18', 'off', '0 : input', '0 : low', '0 : none', '0 : none', '0 : low', '0 : low'; 'C', '19', 'off', '0 : input', '0 : low', '0 : none', '0 : none', '0 : low', '0 : low'; 'C', '20', 'off', '0 : input', '0 : low', '0 : none', '0 : none', '0 : low', '0 : low'; 'C', '21', 'off', '0 : input', '0 : low', '0 : none', '0 : none', '0 : low', '0 : low'; 'C', '22', 'off', '0 : input', '0 : low', '0 : none', '0 : none', '0 : low', '0 : low'; 'C', '23', 'off', '0 : input', '0 : low', '0 : none', '0 : none', '0 : low', '0 : low'; 'C', '24', 'off', '0 : input', '0 : low', '0 : none', '0 : none', '0 : low', '0 : low'; 'C', '25', 'off', '0 : input', '0 : low', '0 : none', '0 : none', '0 : low', '0 : low'; 'C', '26', 'off', '0 : input', '0 : low', '0 : none', '0 : none', '0 : low', '0 : low'; 'C', '27', 'off', '0 : input', '0 : low', '0 : none', '0 : none', '0 : low', '0 : low'; 'C', '28', 'off', '0 : input', '0 : low', '0 : none', '0 : none', '0 : low', '0 : low'; 'C', '29', 'off', '0 : input', '0 : low', '0 : none', '0 : none', '0 : low', '0 : low'; 'C', '30', 'off', '0 : input', '0 : low', '0 : none', '0 : none', '0 : low', '0 : low'; 'C', '31', 'off', '0 : input', '0 : low', '0 : none', '0 : none', '0 : low', '0 : low'; 'D', '0', 'off', '0 : input', '0 : low', '0 : none', '0 : none', '0 : low', '0 : low'; 'D', '1', 'off', '0 : input', '0 : low', '0 : none', '0 : none', '0 : low', '0 : low'; 'D', '2', 'off', '0 : input', '0 : low', '0 : none', '0 : none', '0 : low', '0 : low'; 'D', '3', 'off', '0 : input', '0 : low', '0 : none', '0 : none', '0 : low', '0 : low'; 'D', '4', 'off', '0 : input', '0 : low', '0 : none', '0 : none', '0 : low', '0 : low'; 'D', '5', 'off', '0 : input', '0 : low', '0 : none', '0 : none', '0 : low', '0 : low'; 'D', '6', 'off', '0 : input', '0 : low', '0 : none', '0 : none', '0 : low', '0 : low'; 'D', '7', 'off', '0 : input', '0 : low', '0 : none', '0 : none', '0 : low', '0 : low'; 'D', '8', 'off', '0 : input', '0 : low', '0 : none', '0 : none', '0 : low', '0 : low'; 'D', '9', 'off', '0 : input', '0 : low', '0 : none', '0 : none', '0 : low', '0 : low'; 'D', '10', 'off', '0 : input', '0 : low', '0 : none', '0 : none', '0 : low', '0 : low'; 'D', '11', 'off', '0 : input', '0 : low', '0 : none', '0 : none', '0 : low', '0 : low'; 'D', '12', 'off', '0 : input', '0 : low', '0 : none', '0 : none', '0 : low', '0 : low'; 'D', '13', 'off', '0 : input', '0 : low', '0 : none', '0 : none', '0 : low', '0 : low'; 'D', '14', 'off', '0 : input', '0 : low', '0 : none', '0 : none', '0 : low', '0 : low'; 'D', '15', 'off', '0 : input', '0 : low', '0 : none', '0 : none', '0 : low', '0 : low'; 'D', '16', 'off', '0 : input', '0 : low', '0 : none', '0 : none', '0 : low', '0 : low'; 'D', '17', 'off', '0 : input', '0 : low', '0 : none', '0 : none', '0 : low', '0 : low'; 'D', '18', 'off', '0 : input', '0 : low', '0 : none', '0 : none', '0 : low', '0 : low'; 'D', '19', 'off', '0 : input', '0 : low', '0 : none', '0 : none', '0 : low', '0 : low'; 'D', '20', 'off', '0 : input', '0 : low', '0 : none', '0 : none', '0 : low', '0 : low'; 'D', '21', 'off', '0 : input', '0 : low', '0 : none', '0 : none', '0 : low', '0 : low'; 'D', '22', 'off', '0 : input', '0 : low', '0 : none', '0 : none', '0 : low', '0 : low'; 'D', '23', 'off', '0 : input', '0 : low', '0 : none', '0 : none', '0 : low', '0 : low'; 'D', '24', 'off', '0 : input', '0 : low', '0 : none', '0 : none', '0 : low', '0 : low'; 'D', '25', 'off', '0 : input', '0 : low', '0 : none', '0 : none', '0 : low', '0 : low'; 'D', '26', 'off', '0 : input', '0 : low', '0 : none', '0 : none', '0 : low', '0 : low'; 'D', '27', 'off', '0 : input', '0 : low', '0 : none', '0 : none', '0 : low', '0 : low'; 'D', '28', 'off', '0 : input', '0 : low', '0 : none', '0 : none', '0 : low', '0 : low'; 'D', '29', 'off', '0 : input', '0 : low', '0 : none', '0 : none', '0 : low', '0 : low'; 'D', '30', 'off', '0 : input', '0 : low', '0 : none', '0 : none', '0 : low', '0 : low'; 'D', '31', 'off', '0 : input', '0 : low', '0 : none', '0 : none', '0 : low', '0 : low'; 'E', '0', 'off', '0 : input', '0 : low', '0 : none', '0 : none', '0 : low', '0 : low'; 'E', '1', 'off', '0 : input', '0 : low', '0 : none', '0 : none', '0 : low', '0 : low'; 'E', '2', 'off', '0 : input', '0 : low', '0 : none', '0 : none', '0 : low', '0 : low'; 'E', '3', 'off', '0 : input', '0 : low', '0 : none', '0 : none', '0 : low', '0 : low'; 'E', '4', 'off', '0 : input', '0 : low', '0 : none', '0 : none', '0 : low', '0 : low'; 'E', '5', 'off', '0 : input', '0 : low', '0 : none', '0 : none', '0 : low', '0 : low' }  Param_priority=30  Param_sampleTime=-1
      settings: AttributesFormatString=priority=%<priority>  SourceProductName=Peloton Interface Library
  Event Listener : EventListener  DisableCoverage=on  EventName=reset
  LpTimer_StartStop : MbdLib_LpTimer/LpTimer_StartStop  Priority=130  Param_module=1  Param_action=Start  Param_mode=PWM  Param_period=1000  Param_duty=500  Param_priority=130  Param_sampleTime=-1
      settings: AttributesFormatString=priority=%<priority>  SourceProductName=Peloton Interface Library
  LpTimer_StartStop1 : MbdLib_LpTimer/LpTimer_StartStop  Priority=130  Param_module=2  Param_action=Start  Param_mode=PWM  Param_period=1000  Param_duty=500  Param_priority=130  Param_sampleTime=-1
      settings: AttributesFormatString=priority=%<priority>  SourceProductName=Peloton Interface Library
  PWM_StartStop : MbdLib_Pwm/PWM_StartStop  Priority=120  Param_module=2  Param_ch=1  Param_action=Start  Param_priority=120  Param_sampleTime=-1
      settings: AttributesFormatString=priority=%<priority>  SourceProductName=Peloton Interface Library
  PWM_StartStop1 : MbdLib_Pwm/PWM_StartStop  Priority=120  Param_module=2  Param_ch=2  Param_action=Start  Param_priority=120  Param_sampleTime=-1
      settings: AttributesFormatString=priority=%<priority>  SourceProductName=Peloton Interface Library
  PWM_StartStop2 : MbdLib_Pwm/PWM_StartStop  Priority=120  Param_module=1  Param_ch=1  Param_action=Start  Param_priority=120  Param_sampleTime=-1
      settings: AttributesFormatString=priority=%<priority>  SourceProductName=Peloton Interface Library
  PWM_StartStop3 : MbdLib_Pwm/PWM_StartStop  Priority=120  Param_module=1  Param_ch=2  Param_action=Start  Param_priority=120  Param_sampleTime=-1
      settings: AttributesFormatString=priority=%<priority>  SourceProductName=Peloton Interface Library
  Timer_Config : MbdLib_Timer/Timer_Config  Priority=100  Param_update=1  Param_module=6  Param_step=0  Param_period=LED1_period_cycles  Param_divider=LED1_clock_divider  Param_step0=0  Param_clksrc0=0  Param_period0=LED1_period_cycles  Param_divider0=LED1_clock_divider  Param_step1=-1  Param_clksrc1=0  Param_period1=0  Param_divider1=0  Param_step2=-1  Param_clksrc2=0  Param_period2=0  Param_divider2=0  Param_priority=100  Param_sampleTime=-1
      settings: AttributesFormatString=priority=%<priority>  SourceProductName=Peloton Interface Library
  Timer_Config1 : MbdLib_Timer/Timer_Config  Priority=101  Param_update=1  Param_module=15  Param_step=1  Param_period=LED2_period_cycles  Param_divider=LED2_clock_divider  Param_step0=1  Param_clksrc0=0  Param_period0=LED2_period_cycles  Param_divider0=LED2_clock_divider  Param_step1=-1  Param_clksrc1=0  Param_period1=0  Param_divider1=0  Param_step2=-1  Param_clksrc2=0  Param_period2=0  Param_divider2=0  Param_priority=101  Param_sampleTime=-1
      settings: AttributesFormatString=priority=%<priority>  SourceProductName=Peloton Interface Library
